simulink model "AEB_Level_0"  (R2023b)
settings: Solver=ode1  StartTime=0.0  StopTime=inf  FixedStep=0.001  RelTol=1e-3
settings Model: Creator=varunvaidhiya  LastModifiedBy=varunvaidhiya
settings DebuggingCC: SFUnexpectedBacktrackingDiag=warning  SFNoUnconditionalDefaultTransitionDiag=warning  UnderSpecifiedDimensionMsg=warning

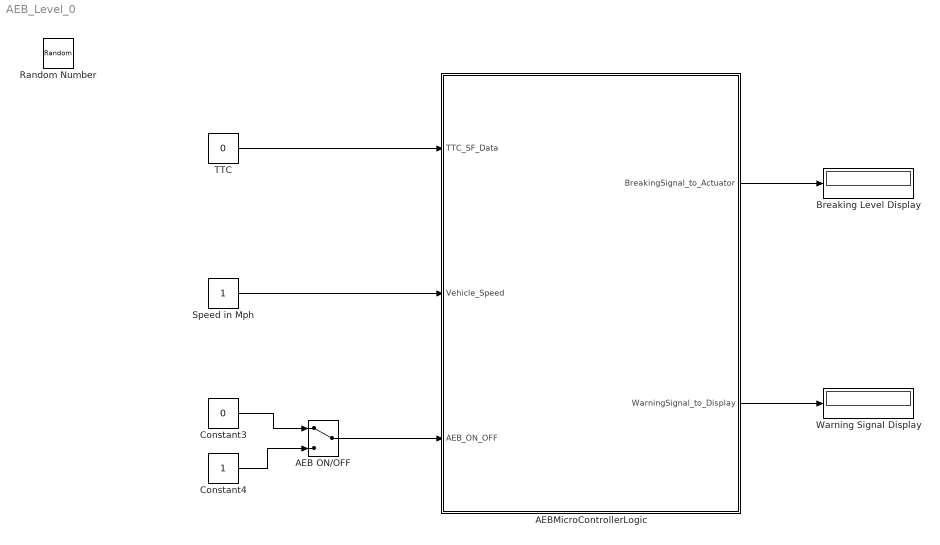
== system AEB_Level_0 ==
  AEB ON/OFF : ManualSwitch
  AEBMicroControllerLogic : Stateflow chart  TreatAsAtomicUnit=on
  Breaking Level Display : Display
  Constant3 : Constant  Value=0  OutDataTypeStr=boolean
  Constant4 : Constant  OutDataTypeStr=boolean
  Speed in Mph : Constant
  TTC : Constant  Value=0  OutDataTypeStr=int32
  Warning Signal Display : Display
  Random Number : RandomNumber  IOType=siggen  SampleTime=0
  wires:
  Constant3/1 -> AEB ON/OFF/1
  Constant4/1 -> AEB ON/OFF/2
  AEB ON/OFF/1 -> AEBMicroControllerLogic/3(AEB_ON_OFF)
  Speed in Mph/1 -> AEBMicroControllerLogic/2(Vehicle_Speed)
  TTC/1 -> AEBMicroControllerLogic/1(TTC_SF_Data)
  AEBMicroControllerLogic/1(BreakingSignal_to_Actuator) -> Breaking Level Display/1
  AEBMicroControllerLogic/2(WarningSignal_to_Display) -> Warning Signal Display/1

== stateflow chart AEB_Level_0/AEBMicroControllerLogic ==
  state AEBControllerAction
    state FCW
      BreakingSignal_to_Actuator=0;
      WarningSignal_to_Display = true;
    state PB1
      BreakingSignal_to_Actuator=1;
      WarningSignal_to_Display = true;
    state PB2
      BreakingSignal_to_Actuator = 2;
      WarningSignal_to_Display =true;
    state FB
      BreakingSignal_to_Actuator = 3;
      WarningSignal_to_Display =true;
    (junction 26) -> FCW [order 1] : [TTC_SF_Data <= 8]
    (junction 26) -> PB1 [order 2] : [TTC_SF_Data <= 4 && TTC_SF_Data > 3]
    (junction 26) -> PB2 [order 3] : [TTC_SF_Data <= 3 &&TTC_SF_Data > 2]
    (junction 26) -> FB [order 4] : [TTC_SF_Data <= 2]
  state Default
    BreakingSignal_to_Actuator = 0;
    WarningSignal_to_Display = false;
  Default -> Default [order 1] : [AEB_ON_OFF == 0]
  (default) -> Default
  FCW -> (junction 47)
  Default -> (junction 38) [order 2]
  (junction 38) -> (junction 26) : [AEB_ON_OFF == 1 && Vehicle_Speed > 0]
  PB1 -> (junction 47)
  PB2 -> (junction 47)
  (junction 47) -> Default [order 1] : [TTC_SF_Data >=8 ]
  (junction 23) -> Default
  FB -> (junction 47)
  (junction 47) -> (junction 23) [order 2] : [AEB_ON_OFF == 0]
  data: TTC_SF_Data input int32; Vehicle_Speed input int32; AEB_ON_OFF input boolean; BreakingSignal_to_Actuator output int32; WarningSignal_to_Display output boolean
